simulink model "Rider_Controls_Control_CAN_Enable"  (R2014b)
settings: configuration reference "Embedded_Configuration" (kept outside this file)
PreLoadFcn:
  | load('Embedded_Config.mat')
PostLoadFcn:
  | c2000demoscallback(1)
model workspace: external: MAT-File C:\Users\Sean\Desktop\Buckeye Current\MagicSimNode\Embedded_Config.mat (data not in the file)
libraries: canmsglib x5, c280xlib x5
settings Model: Creator=The MathWorks Inc.  LastModifiedBy=Sean

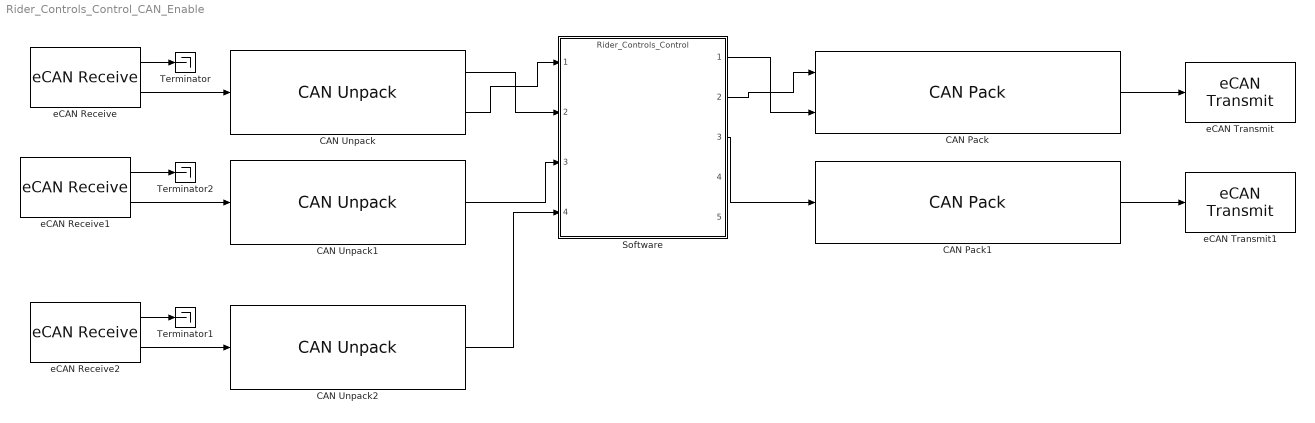
== system Rider_Controls_Control_CAN_Enable ==
  CAN Pack : canmsglib/CAN Pack  CANdbFile=C:\Users\Nathan\Desktop\Git\EmbeddedCoderC2000\Rider_Controls\Rider_Controls_Debug.dbc  MsgList=Control_Ouput  MsgName=Control_Ouput  MsgIDType=Standard (11-bit identifier)  MsgIdentifier=1  MsgLength=8  SignalInfo=Lookup$32$32$1$3$1$0$1$0$-10000$10000$#Motor_Current_percent$0$32$1$3$1$0$1$0$-1000$1000$#  NSignals=2  StartBits=str2num('[int32(32);int32(0)]')  SignalSizes=str2num('[int32(32);int32(32)]')  ByteOrders=str2num('[int32(1);int32(1)]')  DataTypes=str2num('[int32(3);int32(3)]')  MultiplexTypes=str2num('[int32(1);int32(1)]')  MultiplexValues=str2num('[double(0);double(0)]')  Factors=str2num('[double(1);double(1)]')  Offsets=str2num('[double(0);double(0)]')  Minimums=str2num('[double(-10000);double(-1000)]')  Maximums=str2num('[double(10000);double(1000)]')  Remote=off
      settings: DataFormat=CANdb specified signals
  CAN Pack1 : canmsglib/CAN Pack  CANdbFile=C:\Users\Nathan\Desktop\Git\EmbeddedCoderC2000\Rider_Controls\Rider_Controls_Debug.dbc  MsgList=Control_Output3  MsgName=Control_Output3  MsgIDType=Standard (11-bit identifier)  MsgIdentifier=3  MsgLength=8  SignalInfo=Batt_Lookup$0$32$1$3$1$0$1$0$-1000$10000$#  NSignals=1  StartBits=str2num('[int32(0)]')  SignalSizes=str2num('[int32(32)]')  ByteOrders=str2num('[int32(1)]')  DataTypes=str2num('[int32(3)]')  MultiplexTypes=str2num('[int32(1)]')  MultiplexValues=str2num('[double(0)]')  Factors=str2num('[double(1)]')  Offsets=str2num('[double(0)]')  Minimums=str2num('[double(-1000)]')  Maximums=str2num('[double(10000)]')  Remote=off
      settings: DataFormat=CANdb specified signals
  CAN Unpack : canmsglib/CAN Unpack  CANdbFile=C:\Users\Nathan\Desktop\Git\EmbeddedCoderC2000\Rider_Controls\Rider_Controls_Debug.dbc  MsgList=Control_Input  MsgName=Control_Input12  MsgIDType=Standard (11-bit identifier)  MsgIdentifier=0  MsgLength=8  SignalInfo=RPM$32$32$1$3$1$0$1$0$-100000$100000$#Throttle$0$32$1$3$1$0$1$0$-1000$1000$#  NSignals=2  IDPort=off  TimestampPort=off  ErrorPort=off  RemotePort=off  LengthPort=off  StatusPort=off  StartBits=str2num('[int32(32);int32(0)]')  SignalSizes=str2num('[int32(32);int32(32)]')  ByteOrders=str2num('[int32(1);int32(1)]')  DataTypes=str2num('[int32(3);int32(3)]')  MultiplexTypes=str2num('[int32(1);int32(1)]')  MultiplexValues=str2num('[double(0);double(0)]')  Factors=str2num('[double(1);double(1)]')  Offsets=str2num('[double(0);double(0)]')  Minimums=str2num('[double(-100000);double(-1000)]')  Maximums=str2num('[double(100000);double(1000)]')
      settings: DataFormat=CANdb specified signals
  CAN Unpack1 : canmsglib/CAN Unpack  CANdbFile=C:\Users\Nathan\Desktop\Git\EmbeddedCoderC2000\Rider_Controls\Rider_Controls_Debug.dbc  MsgList=Control_Input3  MsgName=Control_Input3  MsgIDType=Standard (11-bit identifier)  MsgIdentifier=2  MsgLength=8  SignalInfo=Batt_Temp$0$32$1$3$1$0$1$0$-10000$10000$#  NSignals=1  IDPort=off  TimestampPort=off  ErrorPort=off  RemotePort=off  LengthPort=off  StatusPort=off  StartBits=str2num('[int32(0)]')  SignalSizes=str2num('[int32(32)]')  ByteOrders=str2num('[int32(1)]')  DataTypes=str2num('[int32(3)]')  MultiplexTypes=str2num('[int32(1)]')  MultiplexValues=str2num('[double(0)]')  Factors=str2num('[double(1)]')  Offsets=str2num('[double(0)]')  Minimums=str2num('[double(-10000)]')  Maximums=str2num('[double(10000)]')
      settings: DataFormat=CANdb specified signals
  CAN Unpack2 : canmsglib/CAN Unpack  CANdbFile=C:\Users\Nathan\Desktop\Git\EmbeddedCoderC2000\Rider_Controls\Rider_Controls_Debug.dbc  MsgList=Control_Input4  MsgName=Control_Input4  MsgIDType=Standard (11-bit identifier)  MsgIdentifier=4  MsgLength=8  SignalInfo=EStop$0$32$1$3$1$0$1$0$-Inf$Inf$#  NSignals=1  IDPort=off  TimestampPort=off  ErrorPort=off  RemotePort=off  LengthPort=off  StatusPort=off  StartBits=str2num('[int32(0)]')  SignalSizes=str2num('[int32(32)]')  ByteOrders=str2num('[int32(1)]')  DataTypes=str2num('[int32(3)]')  MultiplexTypes=str2num('[int32(1)]')  MultiplexValues=str2num('[double(0)]')  Factors=str2num('[double(1)]')  Offsets=str2num('[double(0)]')  Minimums=str2num('[double(-Inf)]')  Maximums=str2num('[double(Inf)]')
      settings: DataFormat=CANdb specified signals
  Software : ModelReference  ModelNameDialog=Rider_Controls_Control.slx  SimulationMode=Normal  ModelReferenceVersion=1.128  CopyOfModelName=Rider_Controls_Control.slx  DefaultDataLogging=on
  Terminator : Terminator
  Terminator1 : Terminator
  Terminator2 : Terminator
  eCAN Receive : c280xlib/eCAN Receive  chipFamily=C280x  useModule=eCAN_A  mailboxNo=0  messageID=0  messageType=Standard (11-bit identifier)  sampleTime=.01  dataType=CAN_MESSAGE_TYPE  initValue=0  outputMessageLength=off  outputMessageTimeStamp=off  postInterrupt=off  interruptLine=0
  eCAN Receive1 : c280xlib/eCAN Receive  chipFamily=C280x  useModule=eCAN_A  mailboxNo=3  messageID=2  messageType=Standard (11-bit identifier)  sampleTime=.01  dataType=CAN_MESSAGE_TYPE  initValue=0  outputMessageLength=off  outputMessageTimeStamp=off  postInterrupt=off  interruptLine=0
  eCAN Receive2 : c280xlib/eCAN Receive  chipFamily=C280x  useModule=eCAN_A  mailboxNo=0  messageID=0  messageType=Standard (11-bit identifier)  sampleTime=.01  dataType=CAN_MESSAGE_TYPE  initValue=0  outputMessageLength=off  outputMessageTimeStamp=off  postInterrupt=off  interruptLine=0
  eCAN Transmit : c280xlib/eCAN Transmit  chipFamily=C280x  useModule=eCAN_A  mailboxNo=1  messageID=1  messageType=Standard (11-bit identifier)  enableBlockingMode=off  postInterrupt=off  interruptLine=0
  eCAN Transmit1 : c280xlib/eCAN Transmit  chipFamily=C280x  useModule=eCAN_A  mailboxNo=4  messageID=3  messageType=Standard (11-bit identifier)  enableBlockingMode=off  postInterrupt=off  interruptLine=0
  wires:
  CAN Pack/1 -> eCAN Transmit/1
  eCAN Receive/2 -> CAN Unpack/1
  eCAN Receive/1 -> Terminator/1
  Software/1 -> CAN Pack/2
  Software/2 -> CAN Pack/1
  CAN Unpack/1 -> Software/2
  CAN Unpack/2 -> Software/1
  CAN Unpack1/1 -> Software/3
  eCAN Receive1/2 -> CAN Unpack1/1
  Software/3 -> CAN Pack1/1
  CAN Pack1/1 -> eCAN Transmit1/1
  eCAN Receive2/2 -> CAN Unpack2/1
  eCAN Receive2/1 -> Terminator1/1
  eCAN Receive1/1 -> Terminator2/1
  CAN Unpack2/1 -> Software/4
